simulink model "OFDM_QAM_Transceiver"  (R2020b)
settings: Solver=VariableStepAuto  StartTime=0.0  StopTime=50  RelTol=1e-3
libraries: commutil2 x2, commblkcod2 x2, commblkintrlv2 x2, commdigbbndam3 x2, commchan3 x1, commrandsrc3 x1, commsink2 x1
settings Model: Creator=charAn  LastModifiedBy=cosorio
settings DataIOCC: ReturnWorkspaceOutputs=off
settings DebuggingCC: ArithmeticOperatorsInVariantConditions=warning
settings SFSimCC: SimUseLocalCustomCode=off  CustomCodeUndefinedFunction=UseInterfaceOnly
settings RTWCC: RTWUseLocalCustomCode=off
settings CodeAppCC: StateflowObjectComments=on

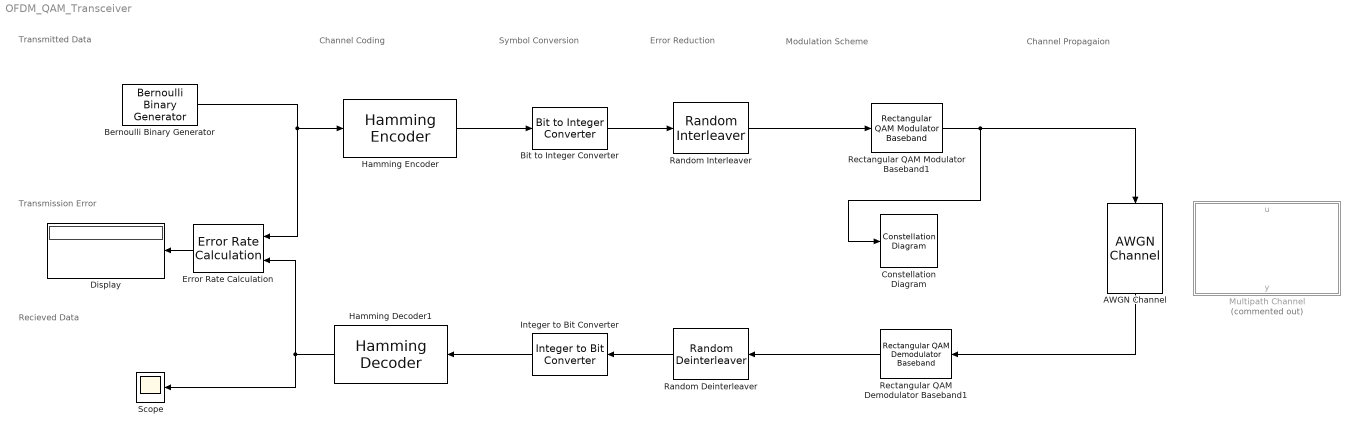
== system OFDM_QAM_Transceiver ==
  note: Transmitted Data
  note: Channel Propagaion
  note: Error Reduction
  note: Symbol Conversion
  note: Channel Coding
  note: Transmission Error
  note: Recieved Data
  note: Modulation Scheme
  AWGN Channel : commchan3/AWGN Channel  InputProcessing=Columns as channels (frame based)  seed=78  noiseMode="Signal to noise ratio  (SNR)"  EbNodB=20  EsNodB=1000  SNRdB=20  bitsPerSym=1  Ps=100  Tsym=1  variance=1
  Bernoulli Binary Generator : commrandsrc3/Bernoulli Binary Generator  ProbabilityOfZero=0.5  SeedSource=Auto  Seed=0  SampleTime=1  SamplesPerFrame=11  OutputDataType=double  SimulateUsing=Interpreted execution
  Bit to Integer Converter : commutil2/Bit to Integer Converter  nbits=3  bitOrder=MSB first  signedOutputValues=Unsigned  outDtype=Inherit via internal rule  outDtypeSigned=Inherit via internal rule
  Constellation Diagram : ConstellationDiagram
  Display : Display
  Error Rate Calculation : commsink2/Error Rate Calculation  N=0  st_delay=0  cp_mode=Entire frame  subframe=[]  PMode=Port  WsName=ErrorVec  RsMode2=off  stop=off  numErr=100  maxBits=1e6
  Hamming Decoder1 : commblkcod2/Hamming Decoder  n=15  k=11
      settings: SourceProductBaseCode=CM
  Hamming Encoder : commblkcod2/Hamming Encoder  n=15  k=11
      settings: SourceProductBaseCode=CM
  Integer to Bit Converter : commutil2/Integer to Bit Converter  nbits=3  signedInputValues=Unsigned  bitOrder=MSB first  outDtype=Inherit via internal rule
  Multipath Channel : MATLAB Function  Commented=on  TreatAsAtomicUnit=on
  Random Deinterleaver : commblkintrlv2/Random Deinterleaver  N=5  seed=12345
      settings: SourceProductBaseCode=CM
  Random Interleaver : commblkintrlv2/Random Interleaver  N=5  seed=12345
      settings: SourceProductBaseCode=CM
  Rectangular QAM Demodulator Baseband1 : commdigbbndam3/Rectangular QAM Demodulator Baseband  M=8  OutType=Integer  DecType=Hard decision  VarSource=Dialog  Variance=1  Dec=Gray  Mapping=[0:15]  PowType=Min. distance between symbols  MinDist=2  AvgPow=1  PeakPow=1  Ph=0  outDtype1=Inherit via internal rule  outDtype2=Inherit via internal rule  derotateFactorWordLen=16  derotateFactorDataTypeStr=Inherit: Same word length as input  derotateFactorLastDataTypeStr=Inherit: Same word length as input  denormFactorWordLen=16  denormFactorDataTypeStr=Inherit: Same word length as input  denormFactorLastDataTypeStr=Inherit: Same word length as input  prodOutWordLen=32  prodOutOverflowMode=Wrap  prodOutRoundingMode=Floor  prodOutOvFlMode=off  prodOutOvFlModeLastStrValue=off  sumWordLen=32
  Rectangular QAM Modulator Baseband1 : commdigbbndam3/Rectangular QAM Modulator Baseband  M=8  InType=Integer  Enc=Gray  Mapping=[0:15]  PowType=Min. distance between symbols  MinDist=2  AvgPow=1  PeakPow=1  Ph=0  outDtype=double  outWordLen=16  outUDDataType=sfix(16)  outFracLenMode=Best precision  outFracLen=15  outDataTypeStr=double  outLastDataTypeStr=double
  Scope : Scope
  wires:
  Random Interleaver/1 -> Rectangular QAM Modulator Baseband1/1
  Hamming Decoder1/1 -> Scope/1, Error Rate Calculation/2
  Error Rate Calculation/1 -> Display/1
  Bernoulli Binary Generator/1 -> Hamming Encoder/1, Error Rate Calculation/1
  Rectangular QAM Demodulator Baseband1/1 -> Random Deinterleaver/1
  Bit to Integer Converter/1 -> Random Interleaver/1
  Integer to Bit Converter/1 -> Hamming Decoder1/1
  Hamming Encoder/1 -> Bit to Integer Converter/1
  Random Deinterleaver/1 -> Integer to Bit Converter/1
  AWGN Channel/1 -> Rectangular QAM Demodulator Baseband1/1
  Rectangular QAM Modulator Baseband1/1 -> Constellation Diagram/1, AWGN Channel/1

== matlab function OFDM_QAM_Transceiver/Multipath Channel ==
  data: u input; y output size=[5,1]
function y = multichannel_revised(u)

persistent isopaths channel
persistent projector projRadiator beaconPlat hydrophone 
persistent array arrayCollector arrayPlat rx


%% Define the Underwater Channel
propSpeed = 1520;
channelDepth = 200;
OperatingFrequency = 37.5e3; 

prf = 1;
pulseWidth = 10e-3;
pulseBandwidth = 1/pulseWidth;
fs = 2*pulseBandwidth;

if isempty(isopaths)
    isopaths = phased.IsoSpeedUnderwaterPaths('ChannelDepth',channelDepth,...
      'NumPathsSource','Property','NumPaths',1,'PropagationSpeed',propSpeed);
end

if isempty(channel)
    channel = phased.MultipathChannel('OperatingFrequency',OperatingFrequency,...
        'SampleRate',fs);
end
    
%% Define the Acoustic Beacon and Passive Array
% wav = phased.RectangularWaveform('PRF',prf,'PulseWidth',pulseWidth,...
%   'SampleRate',fs);

if isempty(projector)
    projector = phased.IsotropicProjector('VoltageResponse',120);
end

if isempty(projRadiator)
    projRadiator = phased.Radiator('Sensor',projector,...
      'PropagationSpeed',propSpeed,'OperatingFrequency',OperatingFrequency);
end

if isempty(beaconPlat)
    beaconPlat = phased.Platform('InitialPosition',[5000; 2000; -199],...
      'Velocity',[0; 0; 0]);
end

if isempty(hydrophone)
    hydrophone = phased.IsotropicHydrophone('VoltageSensitivity',-150);
end

if isempty(array)
    array = phased.ULA('Element',hydrophone,...
      'NumElements',5,'ElementSpacing',propSpeed/OperatingFrequency/2,...
      'ArrayAxis','y');
end

if isempty(arrayCollector)
    arrayCollector = phased.Collector('Sensor',array,...
      'PropagationSpeed',propSpeed,'OperatingFrequency',OperatingFrequency);
end

if isempty(arrayPlat)
    arrayPlat = phased.Platform('InitialPosition',[0; 0; -10],...
      'Velocity',[0; 0; 0]);
end

if isempty(rx)
    rx = phased.ReceiverPreamp(...
        'Gain',20,...
        'NoiseFigure',10,...
        'SampleRate',fs,...
        'SeedSource','Property',...
        'Seed',2007);
end

%% Simulate the Passive Sonar System

x = [u; 1 ;zeros(50+94,1);zeros(50,1) ];

numTransmits = 5;
rxsig = zeros(size(x,1),5,numTransmits);
for i = 1:numTransmits

  % Update array and acoustic beacon positions
  [pos_tx,vel_tx] = beaconPlat(1/prf);
  [pos_rx,vel_rx] = arrayPlat(1/prf);

  % Compute paths between the acoustic beacon and array
  [paths,dop,aloss,rcvang,srcang] = ...
      isopaths(pos_tx,pos_rx,vel_tx,vel_rx,1/prf);

  % Propagate the acoustic beacon waveform
  tsig = projRadiator(x,srcang);
  rsig = channel(tsig,paths,dop,aloss);
  
  % Collect the propagated signal
  rsig = arrayCollector(rsig,rcvang);
  
  % Store the received pulses
  rxsig(:,:,i) = abs(rx(rsig));%original
  %rxsig(:,:,i) = abs(rsig);
  
end
  ytemp = [rxsig(110,end),rxsig(111,end), rxsig(112,end), rxsig(113,end), rxsig(114,end), rxsig(115,end)]';
  ytemp = ytemp - mean(rxsig(:,end));
  ytemp = ytemp /(rxsig(115,end) - mean(rxsig(:,end)));
  y = abs(floor(ytemp(1:5)));
  index = find(y>7);
  y(index) = 7;
end
